simulink model "simulation"  (R2019b)
settings: Solver=VariableStepAuto  StartTime=0.0  StopTime=10.0  RelTol=1e-3
libraries: simulink x2, Solver_SF x1
settings Model: Creator=Lenovo  LastModifiedBy=Lenovo

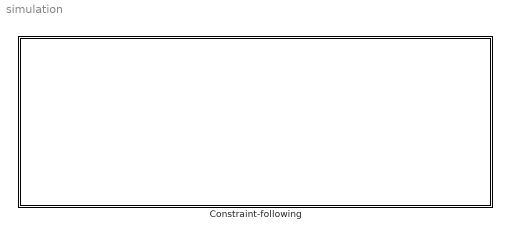
== system simulation ==
  "Constraint-following " : Subsystem

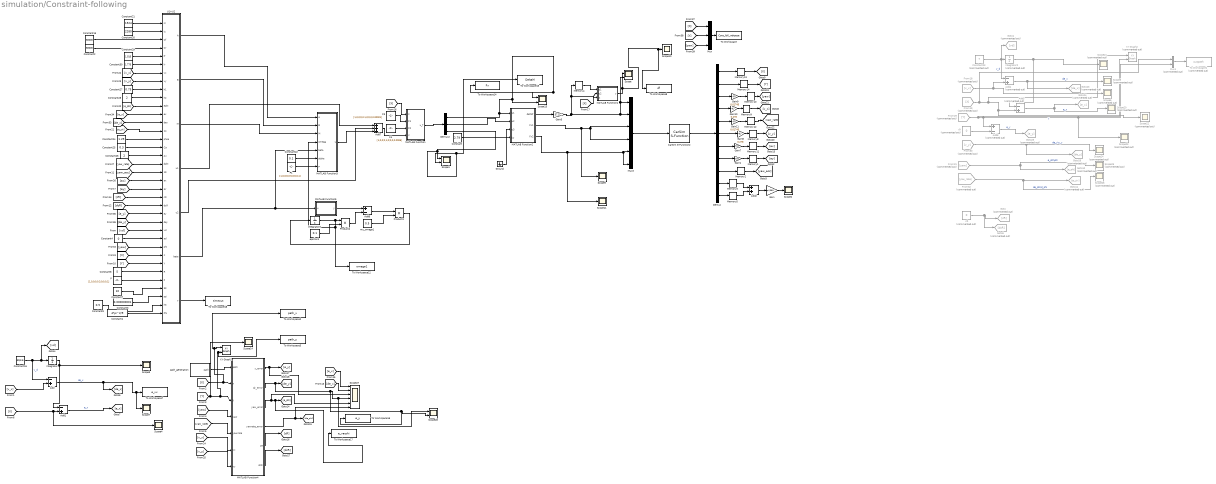
== system simulation/Constraint-following  ==
  Add : Sum  Inputs=-+
  Add1 : Sum  Inputs=-+
  Add2 : Sum
  Add4 : Sum  Commented=on  Inputs=-+
  Add5 : Sum  Commented=on  Inputs=-+
  Add6 : Sum  Inputs=+-
  Add7 : Sum  Inputs=+++
  Add8 : Sum  Commented=on  Inputs=+-
  C3 : Constant  Value=[1,0,0;0,0.1,0;0,0,0.00001]  VectorParams1D=off
  C4 : Constant  Value=[1,0,0;0,1,0;0,0,0.0006]  VectorParams1D=off
  CarSim S-Function2 : Solver_SF/CarSim S-Function  Priority=1  SIMFILE=simfile.sim
  Constant : Constant  Value=2.79
  Constant1 : Constant  Value=4*pi^2/9
  Constant15 : Constant  Value=60000
  Constant16 : Constant  Value=30/3.6
  Constant2 : Constant  Value=60000
  Constant20 : Constant  Value=2280
  Constant21 : Constant  Value=1524
  Constant22 : Constant  Value=0.1
  Constant23 : Constant  Commented=on  Value=7
  Constant24 : Constant  Value=1.29
  Constant25 : Constant  Value=0.3
  Constant26 : Constant  Value=2
  Constant27 : Constant  Value=0.75
  Constant28 : Constant  Value=2
  Constant29 : Constant  Value=1.015
  Constant3 : Constant  Value=0.000000001
  Constant30 : Constant  Value=1.775
  Constant4 : Constant  Value=0
  Constant7 : Constant  Value=10
  Constant8 : Constant  Value=5
  Constant9 : Constant  Value=0.5
  Demux : Demux  Outputs=11
  Demux2 : Demux  Outputs=3
  From18 : From  Commented=on  GotoTag=v_x
  From19 : From  Commented=on  GotoTag=X
  From29 : From  Commented=on  GotoTag=Y
  From30 : From  Commented=on  GotoTag=v_y
  From31 : From  Commented=on  GotoTag=yaw
  From32 : From  Commented=on  GotoTag=yaw_rate
  Gain : Gain  Gain=pi/360
  Gain1 : Gain  Gain=9.8
  Gain10 : Gain  Gain=0.278
  Gain11 : Gain  Gain=0.01745
  Gain5 : Gain  Gain=57.3
  Gain7 : Gain  Gain=9.8
  Gain8 : Gain  Gain=0.278
  Gain9 : Gain  Gain=0.01745
  Goto : Goto  Commented=on  GotoTag=cR
  Goto1 : Goto  Commented=on  GotoTag=vd
  Goto10 : Goto  Commented=on  GotoTag=e_phi
  Goto11 : Goto  Commented=on  GotoTag=de_phi
  Goto23 : Goto  Commented=on  GotoTag=de_x
  Goto24 : Goto  Commented=on  GotoTag=e_x
  Goto25 : Goto  Commented=on  GotoTag=e_y
  Goto26 : Goto  Commented=on  GotoTag=de_y
  Goto5 : Goto  Commented=on  GotoTag=dcR
  Ground : Ground
  Integrator : Integrator
  Integrator2 : Integrator  Commented=on
  Integrator3 : Integrator  InitialCondition=0.5
  MATLAB Function : MATLAB Function  TreatAsAtomicUnit=on
  MATLAB Function1 : MATLAB Function  TreatAsAtomicUnit=on
  MATLAB Function2 : MATLAB Function  TreatAsAtomicUnit=on
  MATLAB Function3 : MATLAB Function  TreatAsAtomicUnit=on
  MATLAB Function4 : MATLAB Function  TreatAsAtomicUnit=on
  MATLAB Function5 : MATLAB Function  TreatAsAtomicUnit=on
  Memory{1..5,8,10..12} (9 alike) : Memory
  Memory13 : Memory  InitialCondition=9.18
  Memory14 : Memory  InitialCondition=20.3
  Memory9 : Memory  InitialCondition=29/3.6
  Mux : Mux  Inputs=3
  Mux1 : Mux  Commented=on  Inputs=2
  Mux3 : Mux  Inputs=6
  P : Constant  Value=[1,0,0;0,0.3,0;0,0,1]  VectorParams1D=off
  P1 : Constant  Value=[1,0,0;0,0.5,0;0,0,1]  VectorParams1D=off
  Product2 : Product
  Product3 : Product
  Scope{,1,13,28} (4 alike) : Scope  NumInputPorts=2
  Scope{2..4,7,9..11,14} (8 alike) : Scope
  Scope{5..6,20..26} (9 alike) : Scope  Commented=on
  Scope27 : Scope  NumInputPorts=6
  To Workspace : ToWorkspace  VariableName=Cons_foll_vehpose  SampleTime=-1
      settings: Save2DSignal=2-D array (concatenate along first dimension)
  To Workspace1 : ToWorkspace  Commented=on  VariableName=outpath  SampleTime=-1
      settings: Save2DSignal=2-D array (concatenate along first dimension)
  To Workspace12 : ToWorkspace  VariableName=omega1  SaveFormat=Timeseries  SampleTime=-1
  To Workspace14 : ToWorkspace  VariableName=Fx  SaveFormat=Timeseries  SampleTime=-1
  To Workspace15 : ToWorkspace  VariableName=DeltaM  SaveFormat=Timeseries  SampleTime=-1
  To Workspace16 : ToWorkspace  VariableName=e_y  SaveFormat=Timeseries  SampleTime=-1
  To Workspace17 : ToWorkspace  VariableName=e_varphi  SaveFormat=Timeseries  SampleTime=-1
  To Workspace18 : ToWorkspace  VariableName=timeout  SaveFormat=Timeseries  SampleTime=-1
  To Workspace2 : ToWorkspace  VariableName=path_x  SampleTime=-1
      settings: Save2DSignal=2-D array (concatenate along first dimension)
  To Workspace3 : ToWorkspace  VariableName=path_y  SampleTime=-1
      settings: Save2DSignal=2-D array (concatenate along first dimension)
  To Workspace7 : ToWorkspace  VariableName=e_vx  SaveFormat=Timeseries  SampleTime=-1
  To Workspace8 : ToWorkspace  VariableName=df  SaveFormat=Timeseries  SampleTime=-1
      settings: Save2DSignal=2-D array (concatenate along first dimension)
  U1+U2 : MATLAB Function  TreatAsAtomicUnit=on
  XY Graph1 : simulink/Sinks/XY Graph  xmin=0  xmax=100  ymin=10  ymax=45  st=-1
  XY Graph2 : simulink/Sinks/XY Graph  Commented=on  xmin=0  xmax=600  ymin=-4  ymax=4  st=-1
  cR : Constant  Commented=on  Value=0
  dY : Constant  Commented=on  Value=0
  epsilon1 : Constant  Value=0.1
  mu_omega1 : Constant  Value=0.5
  path_generation : MATLAB Function  TreatAsAtomicUnit=on
  wires:
  [de_x] -> U1+U2/13(dex)
  Gain1/1 -> Memory1/1
  MATLAB Function4/4(yawrate_error) -> Scope27/6, [de_phi]
  From19/1 -> Mux1/1, XY Graph2/1, Scope22/1, Add5/2
  path_generation/1(path) -> MATLAB Function4/1(path)
  [v_x] -> MATLAB Function4/6(vx)
  Constant27/1 -> U1+U2/9(h1)
  [v_x] -> Add/2
  Memory4/1 -> MATLAB Function1/1(u1)
  [yaw] -> MATLAB Function4/4(yaw)
  MATLAB Function/1(u_f) -> Demux2/1
  From31/1 -> Goto10/1, Scope25/1  "e_phi\\phi"
  [e_x] -> Scope27/1
  C3/1 -> MATLAB Function/2(C1)
  [X] -> MATLAB Function/1(X)
  Add/1 -> [de_x], Scope7/1, To Workspace7/1  "de_x"
  [de_x] -> Scope27/2
  MATLAB Function5/1(y) -> Add6/1
  Constant1/1 -> U1+U2/36(Phi)
  [yaw_rate] -> MATLAB Function4/5(yawrate)
  [Y] -> To Workspace3/1, XY Graph1/2, MATLAB Function4/3(y), Scope14/1
  [v_y] -> MATLAB Function4/7(vy)
  MATLAB Function3/1(u) -> Add7/3
  Constant25/1 -> U1+U2/16(Ca)
  MATLAB Function4/1(y_error) -> Scope27/3, [e_y]
  Constant21/1 -> U1+U2/1(m)
  Constant2/1 -> U1+U2/4(Cr)
  Add8/1 -> Goto25/1  "e_y"
  MATLAB Function4/5(cR) -> [cR]
  U1+U2/1(A) -> MATLAB Function3/1(A)
  Add4/1 -> Goto23/1, Scope5/1  "de_x"
  [e_x] -> U1+U2/12(ex)
  From32/1 -> Goto11/1, Scope26/1  "de_phi\\d_phi"
  [X] -> XY Graph1/1, To Workspace2/1, MATLAB Function4/2(x)
  Memory9/1 -> [v_x]
  epsilon1/1 -> Product2/2
  Memory1/1 -> [ay]
  [e_y] -> U1+U2/24(ey)
  Add7/1 -> MATLAB Function/4(u)
  Constant29/1 -> U1+U2/5(lf)
  [yaw_acc] -> U1+U2/19(ddphi)
  Constant28/1 -> U1+U2/10(h2)
  Demux/5 -> Gain11/1
  [de_y] -> U1+U2/25(dey)
  Demux/9 -> Memory2/1
  Constant24/1 -> U1+U2/15(phoa)
  Demux/1 -> Memory13/1
  Demux/8 -> Gain1/1
  [e_phi] -> U1+U2/11(ephi)
  [dcR] -> U1+U2/23(dcR)
  Constant20/1 -> U1+U2/2(Iz)
  U1+U2/5(u2) -> Add7/2
  Gain11/1 -> Memory12/1
  Constant8/1 -> U1+U2/31(R)
  Product2/1 -> Add6/2
  [X] -> U1+U2/29(X)
  Demux/4 -> Gain10/1
  Add6/1 -> Product3/1
  MATLAB Function2/2(Fx1) -> Scope9/1, Mux3/4, Mux3/3
  [de_phi] -> U1+U2/14(dephi)
  Constant3/1 -> U1+U2/34(psi)
  Constant4/1 -> U1+U2/27(ad)
  Demux2/2 -> MATLAB Function2/2(u2)
  Constant30/1 -> U1+U2/6(lr)
  Demux/6 -> Gain8/1
  Gain8/1 -> Memory8/1
  dY/1 -> Add8/2
  [X] -> MATLAB Function1/3(X)
  MATLAB Function2/3(Fx2) -> Scope11/1, Mux3/5, Mux3/6
  Memory11/1 -> [ax]
  Constant26/1 -> U1+U2/17(Ax)
  U1+U2/2(B) -> MATLAB Function3/2(B)
  Add5/1 -> Goto24/1, Scope20/1  "e_x"
  Memory13/1 -> [X]
  [ay] -> U1+U2/21(ay)
  Gain9/1 -> Memory10/1
  MATLAB Function4/6(dcR) -> [dcR]
  cR/1 -> Goto5/1, Goto/1
  Memory12/1 -> [yaw_rate]
  U1+U2/3(M) -> MATLAB Function3/3(M)
  Gain7/1 -> Memory11/1
  Product3/1 -> Integrator3/1
  From29/1 -> Mux1/2, Scope23/1, Add8/1, XY Graph2/2  "y"
  Gain5/1 -> Mux3/1, Scope/2, Mux3/2, Memory4/1, MATLAB Function1/2(u2)
  From30/1 -> Goto26/1, Scope24/1  "de_y\\v_y"
  Integrator2/1 -> Scope21/1, Add5/1
  Gain10/1 -> Memory9/1
  mu_omega1/1 -> Product3/2
  [yaw] -> U1+U2/28(phi)
  Memory10/1 -> [yaw]
  Constant15/1 -> U1+U2/3(Cf)
  Add1/1 -> [e_x]  "e_x"
  [yaw_rate] -> U1+U2/18(dphi)
  Constant23/1 -> Integrator2/1, Add4/1, Goto1/1  "v_d"
  From18/1 -> Scope6/1, Add4/2
  [cR] -> U1+U2/22(cR)
  Demux/7 -> Gain7/1
  Constant22/1 -> MATLAB Function3/6(alpha)
  P1/1 -> MATLAB Function3/7(P)
  U1+U2/6(beta) -> MATLAB Function5/1(u), MATLAB Function3/5(beta)
  [vd] -> U1+U2/26(vd)
  Constant16/1 -> Add/1, [vd], Integrator/1  "v_d"
  [X] -> Scope4/1, Add1/2
  Integrator/1 -> Scope3/1, Add1/1
  U1+U2/4(u1) -> Add7/1
  Memory8/1 -> [v_y]
  Demux/2 -> Memory14/1
  Constant7/1 -> U1+U2/33(kappa)
  P/1 -> U1+U2/32(P)
  [ax] -> U1+U2/20(ax)
  Constant9/1 -> U1+U2/35(h3)
  [v_y] -> U1+U2/8(vy)
  Memory14/1 -> [Y]
  Memory2/1 -> [yaw_acc]
  [Y] -> U1+U2/30(Y)
  C4/1 -> MATLAB Function/3(C2)
  Demux/3 -> Gain9/1
  [v_x] -> U1+U2/7(vx)
  Integrator3/1 -> MATLAB Function3/4(omega), To Workspace12/1, Product2/1
  MATLAB Function2/1(deltaf) -> Gain5/1
  Constant/1 -> MATLAB Function2/4(lw)
  Mux/1 -> To Workspace/1
  [X] -> Mux/1
  [Y] -> Mux/2
  [yaw] -> Mux/3
  Demux/10 -> Memory3/1
  Demux/11 -> Memory5/1
  Memory5/1 -> Add2/2
  Memory3/1 -> Add2/1
  Add2/1 -> Gain/1
  Gain/1 -> Scope2/1
  MATLAB Function1/1(y) -> To Workspace8/1, Scope10/1, Scope/1
  MATLAB Function4/2(dy_error) -> To Workspace16/1, Scope28/2, Scope28/1, Scope27/4, [de_y]
  MATLAB Function4/3(yaw_error) -> Scope27/5, To Workspace17/1, [e_phi]
  U1+U2/7(timout) -> To Workspace18/1
  Mux1/1 -> To Workspace1/1
  Mux3/1 -> CarSim S-Function2/1
  CarSim S-Function2/1 -> Demux/1
  Demux2/1 -> To Workspace14/1, Scope13/1, Scope13/2, MATLAB Function2/1(u1)
  Demux2/3 -> To Workspace15/1, Scope1/2, Scope1/1
  Ground/1 -> MATLAB Function2/3(u3)

== matlab function simulation/Constraint-following /MATLAB Function1 ==
  data: u1 input; y output; u2 input; X input
function y = fcn(u1,u2,X)
% 直线
%  if (X>80)&&(X<110.5)&&(norm(u2-u1)>0.2)
%     y=0.00001*u2;
% elseif (X>118)&&(X<138)&&(norm(u2-u1)>0.2)
%     y=0.00001*u2;
%     elseif (X>170)&&(X<196)&&(norm(u2-u1)>0.2)
%     y=0.00001*u2;
%     elseif (X>230)&&(X<256)&&(norm(u2-u1)>0.2)
%     y=0.00001*u2;
%     elseif(X>320)&&(X<365.5)&&(norm(u2-u1)>0.2)
%         y=0.00001*u2;
% else
%曲线
if (X>30)&&(X<39)&&(norm(u2-u1)>0.5)
    y=0.005*u2;
    elseif(X>60)&&(X<64.5)&&(norm(u2-u1)>0.5)
        y=0.0005*u2;
else
    y=u2;
end

== matlab function simulation/Constraint-following /MATLAB Function ==
  data: X input; C1 input; C2 input; u input; u_f output
function u_f = fcn(X,C1, C2,u)
%
    u_f=C2*u; 
end

== matlab function simulation/Constraint-following /MATLAB Function2 ==
  data: u1 input; u2 input; u3 input; deltaf output; lw input; Fx1 output; Fx2 output
function [deltaf,Fx1,Fx2] = fcn(u1,u2,u3,lw)
deltaf=u2;
Fx=u1;
DeltaM=u3;
Fx1=(Fx*lw+2*DeltaM)/(4*lw);
Fx2=(Fx*lw-2*DeltaM)/(4*lw);
%定义前左轮为1号，前右胎为2号，后左轮为3号，后右胎为4号；左右轮胎驱动力应不一致才会产生力矩。
end

== matlab function simulation/Constraint-following /MATLAB Function3 ==
  data: A input; B input; M input; omega input; beta input; u output; alpha input; P input

function u  = fcn(A,B,M,omega,beta,alpha,P)

mu=beta*omega;
amu=norm(mu);
if amu>alpha
    gamma=1/amu;
else
    gamma=1/alpha;
    
end
u=-pinv(B)*M*A'/(A*A')/P*gamma*mu*omega;
end

== matlab function simulation/Constraint-following /MATLAB Function4 ==
  data: path input; y_error output; dy_error output; x input; y input; yaw input; yaw_error output; yawrate_error output; yawrate input; vx input; vy input; cR output; dcR output

function [y_error,dy_error,yaw_error,yawrate_error,cR,dcR] = fcn(path,x,y,yaw,yawrate,vx,vy)
%% 轨迹处理 
refPos_x = path(:,1);
refPos_y = path(:,2);
refPos = [refPos_x, refPos_y];
pos=[x,y];
% 计算航向角和曲率
diff_x1 = diff(refPos_x) ;%本质上是一个差分的思想，用后面的减去前面的
diff_x= [diff_x1;diff_x1(end)];
diff_y1 = diff(refPos_y) ;
diff_y = [diff_y1;diff_y1(end)];
derivative1 = gradient(refPos_y) ./ abs(diff_x);              % 一阶导数
derivative2 = del2(refPos_y) ./ abs(diff_x);                  % 二阶导数
derivative3=gradient(del2(refPos_y))./ abs(diff_x); % 三阶导数
refHeading = atan2(diff_y , diff_x);                   % 航向角
refK = abs(derivative2) ./ (1+derivative1.^2).^(3/2);  % 计算曲率
drefK=abs(derivative3+derivative3.*derivative1.^2-3*derivative1.*derivative2.^2)./(1+derivative1.^2).^3; % 计算曲率的导数
%% 首先在参考轨迹上搜索离当前车辆位置最近的点
% 找到距离当前位置最近的一个参考轨迹点的序号
sizeOfrefPos = size(refPos,1);
dist=refPos(:,1);
for i = 1:sizeOfrefPos
    dist(i,1) = norm(refPos(i,:) - pos);   
end
[~,idx] = min(dist); 
% 从该点开始向轨迹前方搜索，找到与预瞄距离最相近的一个轨迹点
     % 从该点开始向轨迹前方搜索，找到与预瞄距离最相近的一个轨迹点
L_steps = 0;           % 参考轨迹上几个相邻点的累计距离
% Ld = Kv*v + Ld0;       % Ld0是预瞄距离的下限值；
Ld =0.5;
while L_steps < Ld && idx < sizeOfrefPos
    L_steps = L_steps + norm(refPos(idx + 1,:) - refPos(idx,:));
    idx = idx+1;
end
idx_target = idx;
% if idx>idx_l
%idx_target = idx;
% else
%     idx_target=idx_l;
% end

%% 计算与预瞄点有关的误差
y_error=y-refPos_y(idx_target);
yaw_error=yaw-refHeading(idx_target);
yawrate_error=yawrate-vx*refK(idx_target);
cR=refK(idx_target);
dy_error=vy*cos(yaw_error)+vx*sin(yaw_error);
dcR=drefK(idx_target);
end

== matlab function simulation/Constraint-following /MATLAB Function5 ==
  data: u input; y output
function y = fcn(u)

y = norm(u);

== matlab function simulation/Constraint-following /U1+U2 ==
  settings: updateMethod=DISCRETE
  data: A output; B output; M output; m input; Iz input; Cf input; Cr input; lf input; lr input; vx input; vy input; h1 input; u1 output; u2 output; h2 input; beta output; ephi input; ex input; dex input; dephi input; phoa input; Ca input; Ax input; dphi input; ddphi input; ax input; ay input; cR input; dcR input; ey input; dey input; vd input; ad input; phi input; X input; Y input; R input; P input; kappa input; psi input; h3 input; Phi input; timout output
function [A,B,M,u1,u2,beta,timout] = fcn(m,Iz,Cf,Cr,lf,lr,vx,vy,h1,h2,ephi,ex,dex,dephi,phoa,Ca,Ax,dphi,ddphi,ax,ay,cR, dcR,ey,dey,vd,ad,phi,X,Y,R,P,kappa,psi,h3,Phi)
%% 建模
tic
M=[m,0,0;0,m,0;0,0,Iz];%quality matrix of vehicle
a1=-2*(Cf+Cr)/vx;
a2=-2*(Cf*lf-Cr*lr)/vx-m*vx;
a3=2*Cf;
a4=-2*(Cf*lf-Cr*lr)/vx;
a5=-2*(Cf*lf^2+Cr*lr^2)/vx;
a6=2*lf*Cf;
dX=vx*sin(phi)-vy*cos(phi);
dY=vx*cos(phi)+vy*sin(phi);
ddX=ax*sin(phi)+vx*dphi*cos(phi)-ay*cos(phi)+vy*dphi*sin(phi);
ddY=ax*cos(phi)-vx*dphi*cos(phi)+ay*sin(phi)+vy*dphi*cos(phi);
B=[1,0,0;0,a3,0;0,a6,1];%take torque into consideration
H=[-0.5*vx^2*phoa*Ca*Ax-0.85*9.8*m;a1*vy+a2*dphi;a4*vy+a5*dphi];%Cause the road slope is 0, only the effect of friction is considered.
dq=[vx;vy;dphi];
%% 横向等式约束
%lp这部分的预瞄距离只能为定常数，因为后续求导未考虑其变化。
lp=0.1*vx;
ep=ey+lp*sin(ephi);
dep=dey+lp*dephi*cos(ephi);
varkappa1=-(cos(ephi)+lp*cR*sin(ephi))*dephi*vx+sin(ephi)*dephi*vy+lp*sin(ephi)*dephi*dphi;
%% 确定系数矩阵

    A= [1,0,0;
        sin(ephi)-lp*cR*cos(ephi),cos(ephi),lp*cos(ephi);
        -cR ,0 ,1];
    c=[vd-h1*ex;-h2*ep;-h3*ephi];
    b=[ad-h1*dex;-h2*dep+varkappa1;vx*dcR-h3*dephi];
   
%% 控制器计算
% L=[1,0,0;0,1,0;0,0,1];
beta=A*dq-c;
T=[39.0384,0,0;0,39.0384,0;0,0,47.07493];%T=sqrtm(M)因为质量不发生变化提前运算完结果
Q=[0.0256,0,0;0,0.0256,0;0,0,0.0209];%同理Q=inv（T）
%u1=pinv(B)*sqrtm(M)*pinv(A/sqrtm(M))*(b-A/M*H);
u1=pinv(B)*T*pinv(A*Q)*(b-A/M*H);
u2=-kappa*pinv(B)*M*A'/(A*A')/P*beta;
timout=toc;
end

== matlab function simulation/Constraint-following /path_generation ==
  data: path output
function path = path_generation()
%% 直线
% shape=2.4;%参数名称，用于参考轨迹生成
% dx1=25;dx2=21.95;%没有任何实际意义，只是参数名称
% dy1=4.05;dy2=5.7;%没有任何实际意义，只是参数名称
% Xs1=27.19;Xs2=56.46;%参数名称
% X_ref=1:0.1:220;%这个点的区间是根据纵向速度（x_dot）来定的，如果速度为10m/s则区间=10*0.1=1
% z1=shape/dx1*(X_ref-Xs1)-shape/2;
% z2=shape/dx2*(X_ref-Xs2)-shape/2;
% Y_ref=dy1/2.*(1+tanh(z1))-dy2/2.*(1+tanh(z2));
% figure(1);
% plot(X_ref, Y_ref,'r--','LineWidth',2);
% hold on;
% % plot(y.signals.values(:,6),y.signals.values(:,5),'g','LineWidth',2);
% hold off;
%% S线
% X_ref=0:0.1:600;
% n=length(X_ref);
% Y_ref=zeros(1,n);
% Y_ref(1,601:1201)=cos(pi/60.*X_ref(1,601:1201))+1;
% Y_ref(1,1202:4201)=2.*cos(pi/60.*(X_ref(1,1202:4201)-120));
% Y_ref(1,4202:4801)=cos(pi/60.*(X_ref(1,4202:4801)))-1;
% plot(X_ref(:,1),Y_ref(:,1));

%% 双移线2
% X_ref=0:0.1:600;
% n=length(X_ref);
% Y_ref=zeros(1,n);
% Y_ref(1,1001:1501)=1.5*sin(pi/50.*(X_ref(1,1001:1501)-125))+1.5;
% Y_ref(1,1502:4501)=3;
% Y_ref(1,4502:5001)=1.5.*cos(pi/50.*(X_ref(1,4502:5001)-450))+1.5;

%% 五次多项式曲线
coefficients = [5.56455900370987e-09,-1.88063163248491e-06,0.000185145086660535,-0.00158567641980212,-0.238324631196854,24.9568568706800];
X_ref=linspace(0, 100, 1000);
Y_ref=polyval(coefficients, X_ref);
%% 路径处理
% 
% 计算Y_ref的一阶导数dy/dx (切线斜率)
Y_prime = gradient(Y_ref, X_ref);

% 计算Y_ref的二阶导数d^2y/dx^2
Y_double_prime = gradient(Y_prime, X_ref);

% 计算切线角度theta
theta = atan(Y_prime);

% 计算曲率kappa
kappa = Y_double_prime ./ (1 + Y_prime.^2).^(3/2);

% 定义一个很大的数值来代替无穷大的曲率半径
large_number = 1e6;

% 计算曲率半径R
R = zeros(size(kappa));
for i = 1:length(kappa)
    if abs(kappa(i)) > 1/large_number
        R(i) = 1 / kappa(i);
    else
        R(i) = large_number; % 当曲率接近零时，设为很大的数值
    end
end

% 组合路径数据
path = [X_ref', Y_ref', theta', R', kappa'];


end
